simulink model "top_model"  (R2017a)
settings: Solver=VariableStepAuto  StartTime=0.0  StopTime=10.0  RelTol=1e-3  EnableMultiTasking=on
PostLoadFcn:
  | load('pcoeffs.mat');
  | load('rcoeffs.mat');
  | 
  | %load('purelongdata.mat');
  | %load('purelongdataval.mat');
  | %load('purelatdata.mat');
  | %load('purelatdataval.mat');
  | load('combineddata.mat');
undefined symbols (not defined in the file): p_Cx1, p_Cy1, p_Dx1, p_Dx2, p_Dx3, p_Dy1, p_Dy2, p_Dy3, p_Ex1, p_Ex2, p_Ex3, p_Ex4, p_Ey1, p_Ey2, p_Ey3, p_Ey4, p_Ey5, p_Kx1, p_Kx2, p_Kx3, p_Ky1, p_Ky2, p_Ky3, p_Ky4, p_Ky5, p_px1, p_px2, p_px3, p_px4, p_py1, p_py2, p_py3, p_py4, r_Bx1, r_Bx2, r_Bx3, r_By1, r_By2, r_By3, r_By4, r_Cx1, r_Cy1, r_Ex1, r_Ex2, r_Ey1, r_Ey2, r_Hx1, r_Hy1, r_Hy2, r_Vy1, r_Vy2, r_Vy3, r_Vy4, r_Vy5, r_Vy6
libraries: simulink_extras x2
settings Model: Creator=The MathWorks, Inc.  LastModifiedBy=Jianming
settings DataIOCC: LimitDataPoints=on
settings OptimizationCC: LifeSpan=inf
settings DebuggingCC: AllowSymbolicDim=off  SFUnexpectedBacktrackingDiag=warning  SFNoUnconditionalDefaultTransitionDiag=warning  SFExecutionAtInitializationDiag=none
settings ModelReferenceCC: PropagateSignalLabelsOutOfModel=off
settings GRTTargetCC: TargetLangStandard=C89/C90 (ANSI)
settings ConfigComp: CovMetricSettings=dw  CovHtmlReporting=on  CovSaveCumulativeToWorkspaceVar=on  CovSaveSingleToWorkspaceVar=on  CovExternalEMLEnable=off

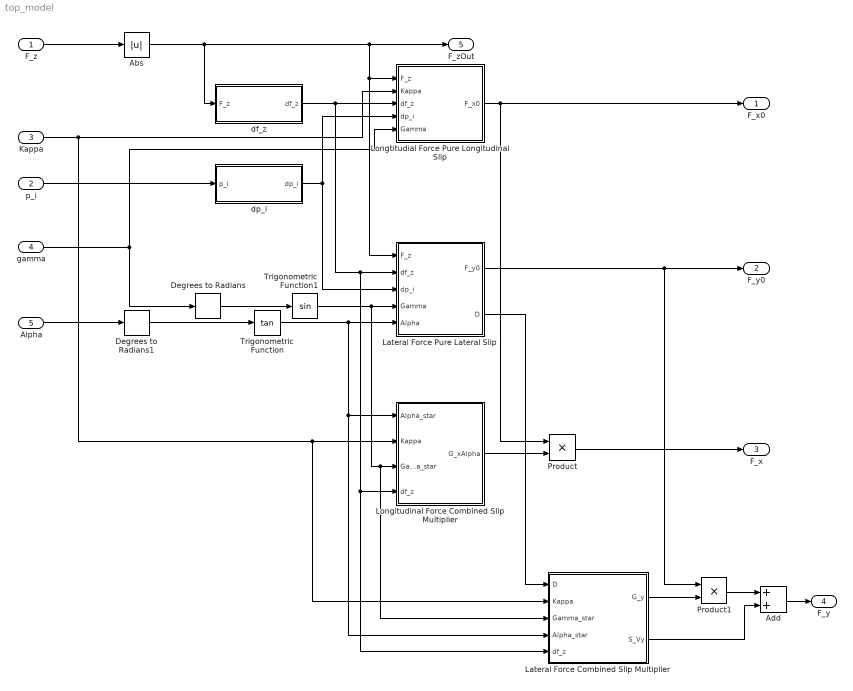
== system top_model ==
  F_z : Inport
  p_i : Inport  Port=2
  Kappa : Inport  Port=3
  gamma : Inport  Port=4
  Alpha : Inport  Port=5
  Abs : Abs
  Add : Sum
  Degrees to Radians : simulink_extras/Transformations/Degrees to Radians
  Degrees to Radians1 : simulink_extras/Transformations/Degrees to Radians
  Lateral Force Combined Slip Multiplier : Subsystem
  Lateral Force Pure Lateral Slip : Subsystem
  Longitudinal Force Combined Slip Multiplier : Subsystem
  Longtitudial Force Pure Longitudinal Slip : Subsystem
  Product : Product
  Product1 : Product
  Trigonometric Function : Trigonometry  Operator=tan
  Trigonometric Function1 : Trigonometry
  df_z : Subsystem
  dp_i : Subsystem
  F_x0 : Outport
  F_y0 : Outport  Port=2
  F_x : Outport  Port=3
  F_y : Outport  Port=4
  F_zOut : Outport  Port=5
  wires:
  Longtitudial Force Pure Longitudinal Slip/1(F_x0) -> Product/1, F_x0/1
  df_z/1(df_z) -> Lateral Force Combined Slip Multiplier/5(df_z), Longitudinal Force Combined Slip Multiplier/4(df_z), Lateral Force Pure Lateral Slip/2(df_z), Longtitudial Force Pure Longitudinal Slip/3(df_z)
  dp_i/1(dp_i) -> Lateral Force Pure Lateral Slip/3(dp_i), Longtitudial Force Pure Longitudinal Slip/4(dp_i)
  gamma/1 -> Longtitudial Force Pure Longitudinal Slip/5(Gamma), Degrees to Radians/1
  Kappa/1 -> Lateral Force Combined Slip Multiplier/2(Kappa), Longitudinal Force Combined Slip Multiplier/2(Kappa), Longtitudial Force Pure Longitudinal Slip/2(Kappa)
  p_i/1 -> dp_i/1(p_i)
  Lateral Force Pure Lateral Slip/1(F_y0) -> Product1/1, F_y0/1
  Alpha/1 -> Degrees to Radians1/1
  Degrees to Radians/1 -> Trigonometric Function1/1
  Degrees to Radians1/1 -> Trigonometric Function/1
  Trigonometric Function/1 -> Lateral Force Combined Slip Multiplier/4(Alpha_star), Longitudinal Force Combined Slip Multiplier/1(Alpha_star), Lateral Force Pure Lateral Slip/5(Alpha)
  Trigonometric Function1/1 -> Lateral Force Combined Slip Multiplier/3(Gamma_star), Longitudinal Force Combined Slip Multiplier/3(Gamma_star), Lateral Force Pure Lateral Slip/4(Gamma)
  F_z/1 -> Abs/1
  Longitudinal Force Combined Slip Multiplier/1(G_xAlpha) -> Product/2
  Product/1 -> F_x/1
  Lateral Force Pure Lateral Slip/2(D) -> Lateral Force Combined Slip Multiplier/1(D)
  Lateral Force Combined Slip Multiplier/1(G_y) -> Product1/2
  Abs/1 -> df_z/1(F_z), F_zOut/1, Lateral Force Pure Lateral Slip/1(F_z), Longtitudial Force Pure Longitudinal Slip/1(F_z)
  Product1/1 -> Add/1
  Lateral Force Combined Slip Multiplier/2(S_Vy) -> Add/2
  Add/1 -> F_y/1

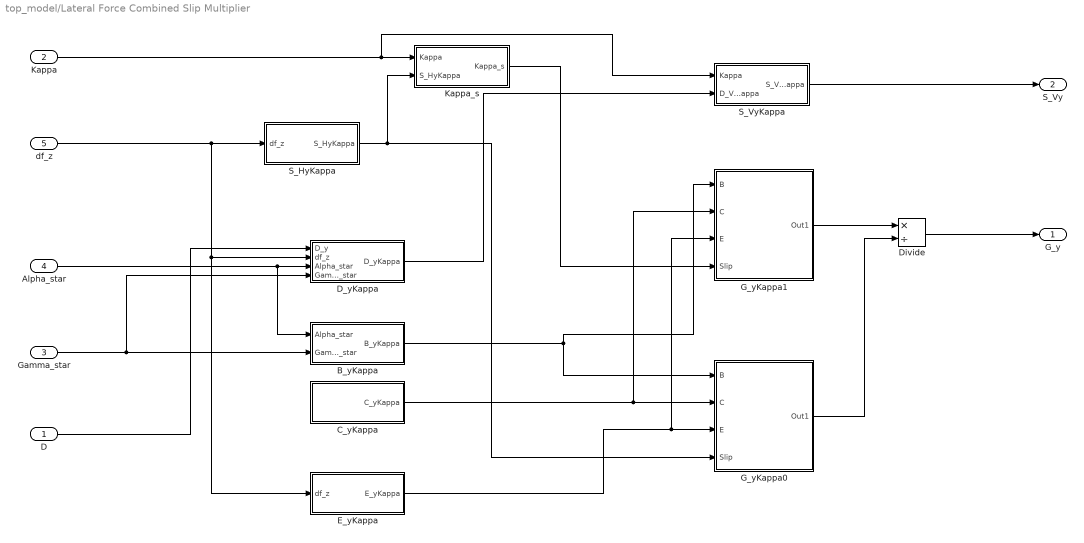
== system top_model/Lateral Force Combined Slip Multiplier ==
  D : Inport
  Kappa : Inport  Port=2
  Gamma_star : Inport  Port=3
  Alpha_star : Inport  Port=4
  df_z : Inport  Port=5
  B_yKappa : Subsystem
  C_yKappa : Subsystem
  D_yKappa : Subsystem
  Divide : Product  Inputs=*/
  E_yKappa : Subsystem
  G_yKappa0 : Subsystem
  G_yKappa1 : Subsystem
  Kappa_s : Subsystem
  S_HyKappa : Subsystem
  S_VyKappa : Subsystem
  G_y : Outport
  S_Vy : Outport  Port=2
  wires:
  G_yKappa1/1(Out1) -> Divide/1
  G_yKappa0/1(Out1) -> Divide/2
  S_VyKappa/1(S_VyKappa) -> S_Vy/1
  Divide/1 -> G_y/1
  Kappa/1 -> S_VyKappa/1(Kappa), Kappa_s/1(Kappa)
  S_HyKappa/1(S_HyKappa) -> Kappa_s/2(S_HyKappa), G_yKappa0/4(Slip)
  df_z/1 -> E_yKappa/1(df_z), D_yKappa/2(df_z), S_HyKappa/1(df_z)
  Kappa_s/1(Kappa_s) -> G_yKappa1/4(Slip)
  C_yKappa/1(C_yKappa) -> G_yKappa1/2(C), G_yKappa0/2(C)
  E_yKappa/1(E_yKappa) -> G_yKappa1/3(E), G_yKappa0/3(E)
  D/1 -> D_yKappa/1(D_y)
  Alpha_star/1 -> B_yKappa/1(Alpha_star), D_yKappa/3(Alpha_star)
  Gamma_star/1 -> D_yKappa/4(Gamma_star), B_yKappa/2(Gamma_star)
  D_yKappa/1(D_yKappa) -> S_VyKappa/2(D_VyKappa)
  B_yKappa/1(B_yKappa) -> G_yKappa1/1(B), G_yKappa0/1(B)

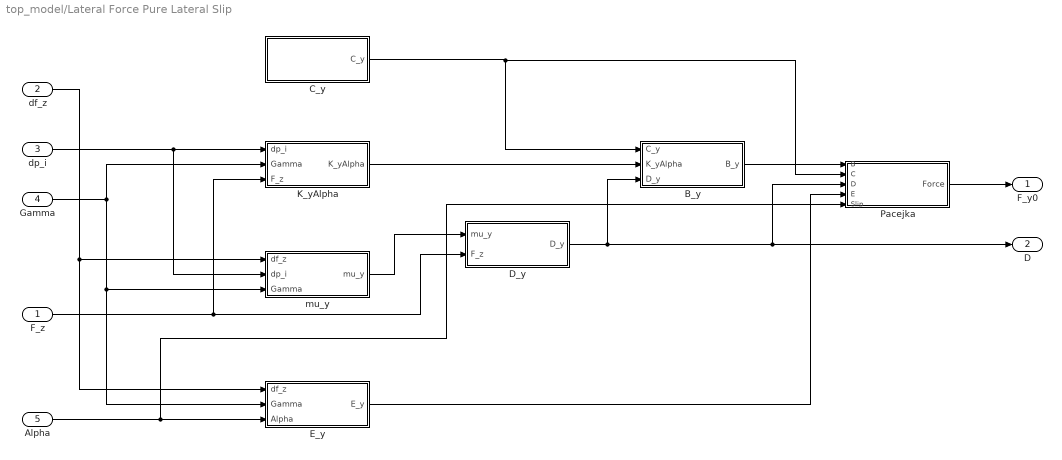
== system top_model/Lateral Force Pure Lateral Slip ==
  F_z : Inport
  df_z : Inport  Port=2
  dp_i : Inport  Port=3
  Gamma : Inport  Port=4
  Alpha : Inport  Port=5
  B_y : Subsystem
  C_y : Subsystem
  D_y : Subsystem
  E_y : Subsystem
  K_yAlpha : Subsystem
  Pacejka : Subsystem
  mu_y : Subsystem
  F_y0 : Outport
  D : Outport  Port=2
  wires:
  K_yAlpha/1(K_yAlpha) -> B_y/2(K_yAlpha)
  Pacejka/1(Force) -> F_y0/1
  D_y/1(D_y) -> D/1, Pacejka/3(D), B_y/3(D_y)
  C_y/1(C_y) -> Pacejka/2(C), B_y/1(C_y)
  B_y/1(B_y) -> Pacejka/1(B)
  E_y/1(E_y) -> Pacejka/4(E)
  mu_y/1(mu_y) -> D_y/1(mu_y)
  F_z/1 -> K_yAlpha/3(F_z), D_y/2(F_z)
  Alpha/1 -> E_y/3(Alpha), Pacejka/5("Slip ")
  df_z/1 -> E_y/1(df_z), mu_y/1(df_z)
  dp_i/1 -> mu_y/2(dp_i), K_yAlpha/1(dp_i)
  Gamma/1 -> E_y/2(Gamma), mu_y/3(Gamma), K_yAlpha/2(Gamma)

== system top_model/Longitudinal Force Combined Slip Multiplier ==
  Alpha_star : Inport
  Kappa : Inport  Port=2
  Gamma_star : Inport  Port=3
  df_z : Inport  Port=4
  Alpha_s : Subsystem
  B_xAlpha : Subsystem
  C_xAlpha : Subsystem
  Divide : Product  Inputs=*/
  E_xAlpha : Subsystem
  G_xAlpha0 : Subsystem
  G_xAlpha2 : Subsystem
  S_HxAlpha : Subsystem
  G_xAlpha : Outport
  wires:
  Alpha_star/1 -> Alpha_s/1(Alpha_star)
  S_HxAlpha/1(S_HxAlpha) -> G_xAlpha0/4(Slip), Alpha_s/2(S_HxAlpha)
  df_z/1 -> E_xAlpha/1(df_z)
  Kappa/1 -> B_xAlpha/2(Kappa)
  Gamma_star/1 -> B_xAlpha/1(Gamma_star)
  B_xAlpha/1(B_xAlpha) -> G_xAlpha0/1(B), G_xAlpha2/1(B)
  C_xAlpha/1(C_xAlpha) -> G_xAlpha0/2(C), G_xAlpha2/2(C)
  E_xAlpha/1(E_xAlpha) -> G_xAlpha0/3(E), G_xAlpha2/3(E)
  Alpha_s/1(Alpha_s) -> G_xAlpha2/4(Slip)
  G_xAlpha2/1(Out1) -> Divide/1
  G_xAlpha0/1(Out1) -> Divide/2
  Divide/1 -> G_xAlpha/1

== system top_model/Longtitudial Force Pure Longitudinal Slip ==
  F_z : Inport
  Kappa : Inport  Port=2
  df_z : Inport  Port=3
  dp_i : Inport  Port=4
  Gamma : Inport  Port=5
  B_x : Subsystem
  "C_x " : Subsystem
  D_x : Subsystem
  E_x : Subsystem
  K_xKappa : Subsystem
  Pacejka : Subsystem
  mu_x : Subsystem
  F_x0 : Outport
  wires:
  mu_x/1(mu_x) -> D_x/2(mu_x)
  F_z/1 -> K_xKappa/1(F_z), D_x/1(F_z)
  D_x/1(D_x) -> Pacejka/3(D), B_x/3(D_x)
  "C_x "/1(C_x) -> Pacejka/2(C), B_x/1(C_x)
  K_xKappa/1(K_xKappa) -> B_x/2(K_xKappa)
  E_x/1(E_x) -> Pacejka/4(E)
  B_x/1(B_x) -> Pacejka/1(B)
  Pacejka/1(Force) -> F_x0/1
  df_z/1 -> K_xKappa/2(df_z), E_x/1(df_z), mu_x/1(df_z)
  dp_i/1 -> K_xKappa/3(dp_i), mu_x/2(dp_i)
  Gamma/1 -> mu_x/3(Gamma)
  Kappa/1 -> E_x/2("kappa "), Pacejka/5("Slip ")

== system top_model/df_z ==
  F_z : Inport
  Divide : Product  Inputs=*/
  F_z0 : Constant  Value=250 * 4.448
  Subtract : Sum  Inputs=+-
  df_z : Outport
  wires:
  F_z/1 -> Subtract/1
  Subtract/1 -> Divide/1
  F_z0/1 -> Divide/2, Subtract/2
  Divide/1 -> df_z/1

== system top_model/dp_i ==
  p_i : Inport
  Divide : Product  Inputs=*/
  Subtract : Sum  Inputs=+-
  p_i0 : Constant  Value=12 * 6.89476
  dp_i : Outport
  wires:
  p_i/1 -> Subtract/1
  Subtract/1 -> Divide/1
  Divide/1 -> dp_i/1
  p_i0/1 -> Divide/2, Subtract/2

== system top_model/Lateral Force Combined Slip Multiplier/B_yKappa ==
  Alpha_star : Inport
  Gamma_star : Inport  Port=2
  Add : Sum
  Constant : Constant  Value=r_By1
  Constant1 : Constant  Value=r_By2
  Constant2 : Constant  Value=r_By3
  Constant3 : Constant  Value=r_By4
  Cos : Trigonometry  Operator=cos
  Product : Product
  Product1 : Product  Inputs=3
  Product2 : Product
  Subtract : Sum  Inputs=+-
  atan : Trigonometry  Operator=atan
  B_yKappa : Outport
  wires:
  Alpha_star/1 -> Subtract/1
  Constant2/1 -> Subtract/2
  Subtract/1 -> Product/2
  Constant1/1 -> Product/1
  Product/1 -> atan/1
  atan/1 -> Cos/1
  Gamma_star/1 -> Product1/2, Product1/1
  Constant3/1 -> Product1/3
  Product1/1 -> Add/2
  Constant/1 -> Add/1
  Cos/1 -> Product2/1
  Add/1 -> Product2/2
  Product2/1 -> B_yKappa/1

== system top_model/Lateral Force Combined Slip Multiplier/C_yKappa ==
  Constant : Constant  Value=r_Cy1
  C_yKappa : Outport
  wires:
  Constant/1 -> C_yKappa/1

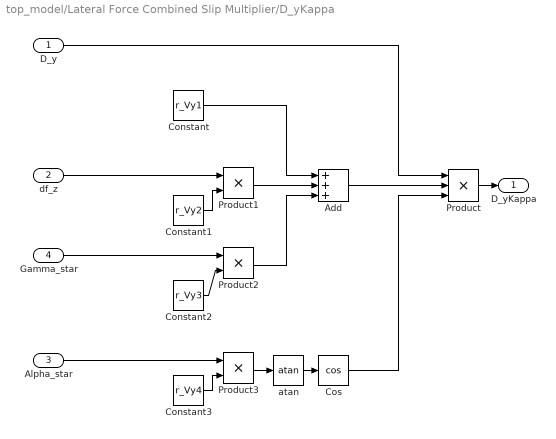
== system top_model/Lateral Force Combined Slip Multiplier/D_yKappa ==
  D_y : Inport
  df_z : Inport  Port=2
  Alpha_star : Inport  Port=3
  Gamma_star : Inport  Port=4
  Add : Sum  Inputs=3
  Constant : Constant  Value=r_Vy1
  Constant1 : Constant  Value=r_Vy2
  Constant2 : Constant  Value=r_Vy3
  Constant3 : Constant  Value=r_Vy4
  Cos : Trigonometry  Operator=cos
  Product : Product  Inputs=3
  Product1 : Product
  Product2 : Product
  Product3 : Product
  atan : Trigonometry  Operator=atan
  D_yKappa : Outport
  wires:
  Product/1 -> D_yKappa/1
  df_z/1 -> Product1/1
  Constant1/1 -> Product1/2
  Constant2/1 -> Product2/2
  Gamma_star/1 -> Product2/1
  Alpha_star/1 -> Product3/1
  Constant3/1 -> Product3/2
  Product3/1 -> atan/1
  atan/1 -> Cos/1
  Constant/1 -> Add/1
  Product1/1 -> Add/2
  Product2/1 -> Add/3
  Add/1 -> Product/2
  Cos/1 -> Product/3
  D_y/1 -> Product/1

== system top_model/Lateral Force Combined Slip Multiplier/E_yKappa ==
  df_z : Inport
  Add : Sum
  Constant : Constant  Value=r_Ey1
  Constant1 : Constant  Value=r_Ey2
  Constant2 : Constant
  Min : MinMax  Inputs=2
  Product : Product
  E_yKappa : Outport
  wires:
  df_z/1 -> Product/1
  Constant1/1 -> Product/2
  Product/1 -> Add/2
  Constant/1 -> Add/1
  Add/1 -> Min/1
  Constant2/1 -> Min/2
  Min/1 -> E_yKappa/1

== system top_model/Lateral Force Combined Slip Multiplier/G_yKappa0 ==
  B : Inport
  C : Inport  Port=2
  E : Inport  Port=3
  Slip : Inport  Port=4
  Cos : Trigonometry  Operator=cos
  Product : Product
  Product1 : Product
  Product2 : Product
  Subtract : Sum  Inputs=+-
  Subtract1 : Sum  Inputs=+-
  atan : Trigonometry  Operator=atan
  atan1 : Trigonometry  Operator=atan
  Out1 : Outport
  wires:
  B/1 -> Product/2
  Slip/1 -> Product/1
  Product/1 -> Subtract1/1, Subtract/1, atan/1
  atan/1 -> Subtract/2
  Subtract/1 -> Product1/1
  E/1 -> Product1/2
  Product1/1 -> Subtract1/2
  Subtract1/1 -> atan1/1
  atan1/1 -> Product2/1
  C/1 -> Product2/2
  Product2/1 -> Cos/1
  Cos/1 -> Out1/1

== system top_model/Lateral Force Combined Slip Multiplier/G_yKappa1 ==
  B : Inport
  C : Inport  Port=2
  E : Inport  Port=3
  Slip : Inport  Port=4
  Cos : Trigonometry  Operator=cos
  Product : Product
  Product1 : Product
  Product2 : Product
  Subtract : Sum  Inputs=+-
  Subtract1 : Sum  Inputs=+-
  atan : Trigonometry  Operator=atan
  atan1 : Trigonometry  Operator=atan
  Out1 : Outport
  wires:
  B/1 -> Product/2
  Slip/1 -> Product/1
  Product/1 -> Subtract1/1, Subtract/1, atan/1
  atan/1 -> Subtract/2
  Subtract/1 -> Product1/1
  E/1 -> Product1/2
  Product1/1 -> Subtract1/2
  Subtract1/1 -> atan1/1
  atan1/1 -> Product2/1
  C/1 -> Product2/2
  Product2/1 -> Cos/1
  Cos/1 -> Out1/1

== system top_model/Lateral Force Combined Slip Multiplier/Kappa_s ==
  Kappa : Inport
  S_HyKappa : Inport  Port=2
  Add : Sum
  Kappa_s : Outport
  wires:
  Kappa/1 -> Add/1
  S_HyKappa/1 -> Add/2
  Add/1 -> Kappa_s/1

== system top_model/Lateral Force Combined Slip Multiplier/S_HyKappa ==
  df_z : Inport
  Add : Sum
  Constant : Constant  Value=r_Hy1
  Constant1 : Constant  Value=r_Hy2
  Product : Product
  S_HyKappa : Outport
  wires:
  df_z/1 -> Product/1
  Constant1/1 -> Product/2
  Product/1 -> Add/2
  Constant/1 -> Add/1
  Add/1 -> S_HyKappa/1

== system top_model/Lateral Force Combined Slip Multiplier/S_VyKappa ==
  Kappa : Inport
  D_VyKappa : Inport  Port=2
  Constant : Constant  Value=r_Vy5
  Constant1 : Constant  Value=r_Vy6
  Product : Product
  Product1 : Product
  Product2 : Product
  Sin : Trigonometry
  atan : Trigonometry  Operator=atan
  S_VyKappa : Outport
  wires:
  Kappa/1 -> Product/1
  Constant1/1 -> Product/2
  Product/1 -> atan/1
  atan/1 -> Product1/2
  Constant/1 -> Product1/1
  Product1/1 -> Sin/1
  Sin/1 -> Product2/1
  D_VyKappa/1 -> Product2/2
  Product2/1 -> S_VyKappa/1

== system top_model/Lateral Force Pure Lateral Slip/B_y ==
  C_y : Inport
  K_yAlpha : Inport  Port=2
  D_y : Inport  Port=3
  Add : Sum
  Divide : Product  Inputs=*/
  Product : Product
  "epsilon " : Constant  Value=0.001
  B_y : Outport
  wires:
  C_y/1 -> Product/1
  D_y/1 -> Product/2
  Product/1 -> Add/1
  "epsilon "/1 -> Add/2
  K_yAlpha/1 -> Divide/1
  Add/1 -> Divide/2
  Divide/1 -> B_y/1

== system top_model/Lateral Force Pure Lateral Slip/C_y ==
  Constant : Constant  Value=p_Cy1
  Constant1 : Constant  Value=0
  Min : MinMax  Function=max  Inputs=2
  C_y : Outport
  wires:
  Constant/1 -> Min/1
  Constant1/1 -> Min/2
  Min/1 -> C_y/1

== system top_model/Lateral Force Pure Lateral Slip/D_y ==
  mu_y : Inport
  F_z : Inport  Port=2
  Constant : Constant  Value=-1000000
  Min : MinMax  Function=max  Inputs=2
  Product : Product
  D_y : Outport
  wires:
  mu_y/1 -> Product/1
  F_z/1 -> Product/2
  Min/1 -> D_y/1
  Product/1 -> Min/1
  Constant/1 -> Min/2

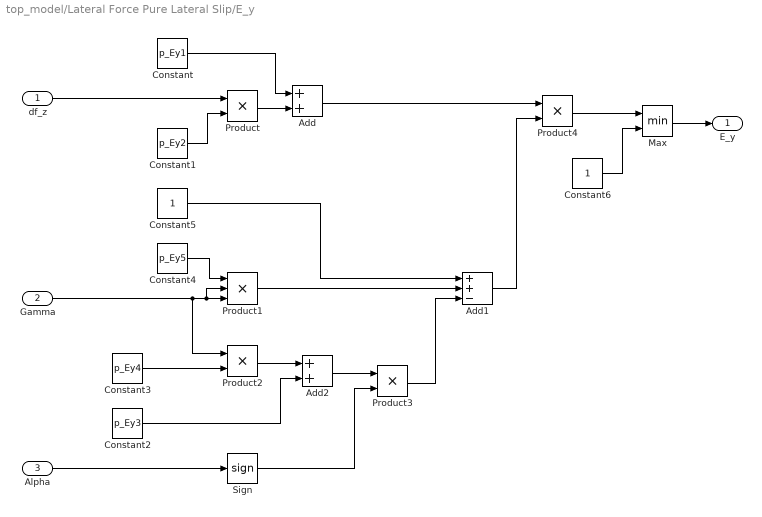
== system top_model/Lateral Force Pure Lateral Slip/E_y ==
  df_z : Inport
  Gamma : Inport  Port=2
  Alpha : Inport  Port=3
  Add : Sum
  Add1 : Sum  Inputs=++-
  Add2 : Sum
  Constant : Constant  Value=p_Ey1
  Constant1 : Constant  Value=p_Ey2
  Constant2 : Constant  Value=p_Ey3
  Constant3 : Constant  Value=p_Ey4
  Constant4 : Constant  Value=p_Ey5
  Constant5 : Constant
  Constant6 : Constant
  Max : MinMax  Inputs=2
  Product{,2..4} (4 alike) : Product
  Product1 : Product  Inputs=3
  Sign : Signum
  E_y : Outport
  wires:
  df_z/1 -> Product/1
  Constant1/1 -> Product/2
  Product/1 -> Add/2
  Constant/1 -> Add/1
  Constant4/1 -> Product1/1
  Gamma/1 -> Product2/1, Product1/2, Product1/3
  Product1/1 -> Add1/2
  Constant5/1 -> Add1/1
  Constant3/1 -> Product2/2
  Product2/1 -> Add2/1
  Constant2/1 -> Add2/2
  Add2/1 -> Product3/1
  Alpha/1 -> Sign/1
  Sign/1 -> Product3/2
  Product3/1 -> Add1/3
  Add/1 -> Product4/1
  Add1/1 -> Product4/2
  Product4/1 -> Max/1
  Constant6/1 -> Max/2
  Max/1 -> E_y/1

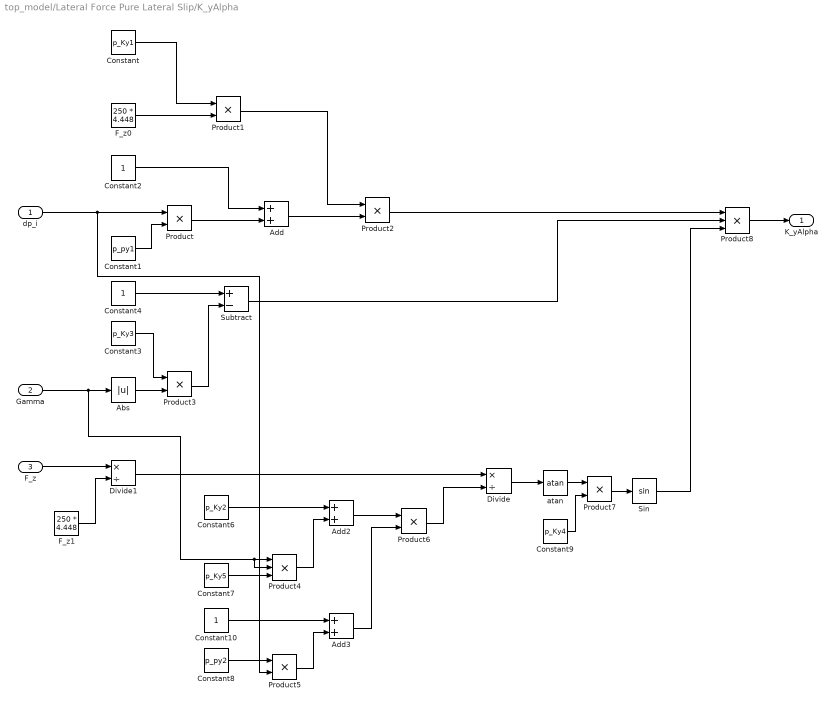
== system top_model/Lateral Force Pure Lateral Slip/K_yAlpha ==
  dp_i : Inport
  Gamma : Inport  Port=2
  F_z : Inport  Port=3
  Abs : Abs
  Add : Sum
  Add2 : Sum
  Add3 : Sum
  Constant : Constant  Value=p_Ky1
  Constant1 : Constant  Value=p_py1
  Constant10 : Constant
  Constant2 : Constant
  Constant3 : Constant  Value=p_Ky3
  Constant4 : Constant
  Constant6 : Constant  Value=p_Ky2
  Constant7 : Constant  Value=p_Ky5
  Constant8 : Constant  Value=p_py2
  Constant9 : Constant  Value=p_Ky4
  Divide : Product  Inputs=*/
  Divide1 : Product  Inputs=*/
  F_z0 : Constant  Value=250 * 4.448
  F_z1 : Constant  Value=250 * 4.448
  Product{,1..3,5..7} (7 alike) : Product
  Product4 : Product  Inputs=3
  Product8 : Product  Inputs=3
  Sin : Trigonometry
  Subtract : Sum  Inputs=+-
  atan : Trigonometry  Operator=atan
  K_yAlpha : Outport
  wires:
  dp_i/1 -> Product5/2, Product/1
  Constant1/1 -> Product/2
  Product/1 -> Add/2
  Constant2/1 -> Add/1
  F_z0/1 -> Product1/2
  Constant/1 -> Product1/1
  Add/1 -> Product2/2
  Product1/1 -> Product2/1
  Constant4/1 -> Subtract/1
  Gamma/1 -> Product4/1, Product4/2, Abs/1
  Constant3/1 -> Product3/1
  Product3/1 -> Subtract/2
  Abs/1 -> Product3/2
  Constant7/1 -> Product4/3
  Product4/1 -> Add2/2
  Constant6/1 -> Add2/1
  Constant8/1 -> Product5/1
  Add2/1 -> Product6/1
  Product6/1 -> Divide/2
  Divide1/1 -> Divide/1
  Divide/1 -> atan/1
  atan/1 -> Product7/1
  Constant9/1 -> Product7/2
  Product7/1 -> Sin/1
  Product2/1 -> Product8/1
  Subtract/1 -> Product8/2
  Sin/1 -> Product8/3
  Product8/1 -> K_yAlpha/1
  Constant10/1 -> Add3/1
  Product5/1 -> Add3/2
  Add3/1 -> Product6/2
  F_z1/1 -> Divide1/2
  F_z/1 -> Divide1/1

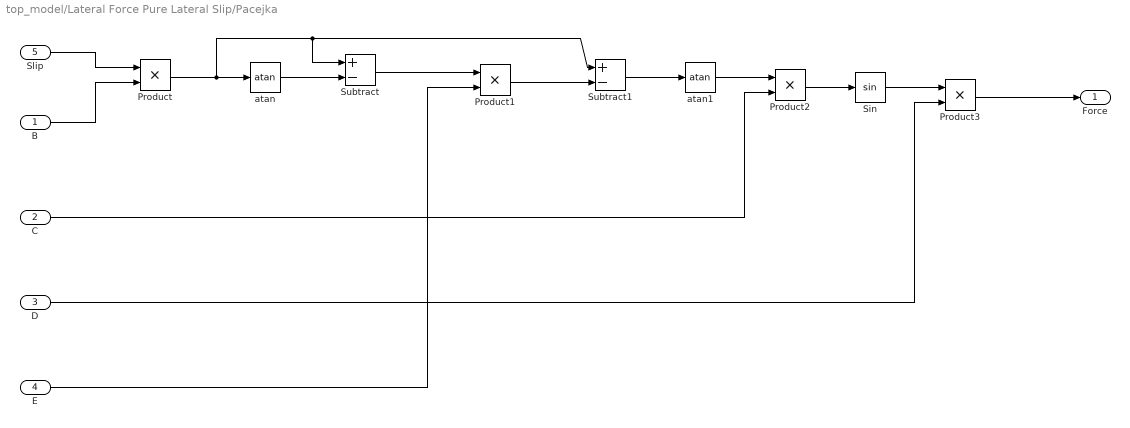
== system top_model/Lateral Force Pure Lateral Slip/Pacejka ==
  B : Inport
  C : Inport  Port=2
  D : Inport  Port=3
  E : Inport  Port=4
  "Slip " : Inport  Port=5
  Product{,1..3} (4 alike) : Product
  Sin : Trigonometry
  Subtract : Sum  Inputs=+-
  Subtract1 : Sum  Inputs=+-
  atan : Trigonometry  Operator=atan
  atan1 : Trigonometry  Operator=atan
  Force : Outport
  wires:
  "Slip "/1 -> Product/1
  B/1 -> Product/2
  Product/1 -> Subtract1/1, Subtract/1, atan/1
  atan/1 -> Subtract/2
  Subtract/1 -> Product1/1
  E/1 -> Product1/2
  Product1/1 -> Subtract1/2
  Subtract1/1 -> atan1/1
  atan1/1 -> Product2/1
  C/1 -> Product2/2
  Product2/1 -> Sin/1
  Sin/1 -> Product3/1
  D/1 -> Product3/2
  Product3/1 -> Force/1

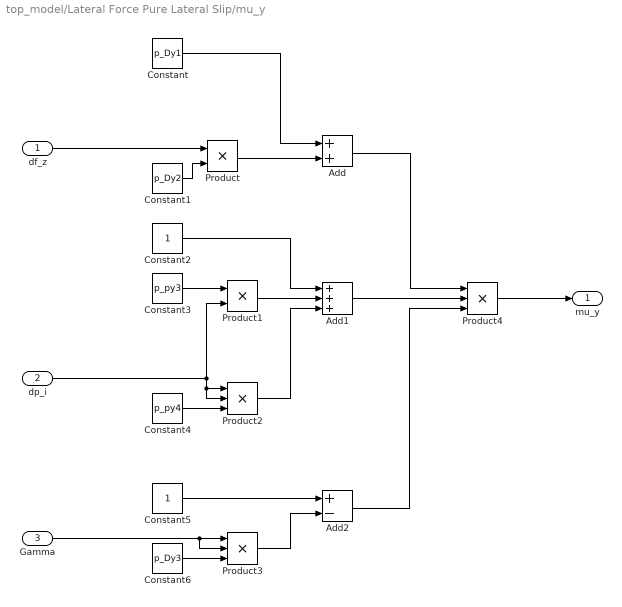
== system top_model/Lateral Force Pure Lateral Slip/mu_y ==
  df_z : Inport
  dp_i : Inport  Port=2
  Gamma : Inport  Port=3
  Add : Sum
  Add1 : Sum  Inputs=3
  Add2 : Sum  Inputs=+-
  Constant : Constant  Value=p_Dy1
  Constant1 : Constant  Value=p_Dy2
  Constant2 : Constant
  Constant3 : Constant  Value=p_py3
  Constant4 : Constant  Value=p_py4
  Constant5 : Constant
  Constant6 : Constant  Value=p_Dy3
  Product : Product
  Product1 : Product
  Product2 : Product  Inputs=3
  Product3 : Product  Inputs=3
  Product4 : Product  Inputs=3
  mu_y : Outport
  wires:
  df_z/1 -> Product/1
  Constant1/1 -> Product/2
  Product/1 -> Add/2
  Constant/1 -> Add/1
  Constant3/1 -> Product1/1
  dp_i/1 -> Product2/1, Product2/2, Product1/2
  Constant4/1 -> Product2/3
  Product1/1 -> Add1/2
  Constant2/1 -> Add1/1
  Product2/1 -> Add1/3
  Gamma/1 -> Product3/2, Product3/1
  Constant6/1 -> Product3/3
  Constant5/1 -> Add2/1
  Product3/1 -> Add2/2
  Add1/1 -> Product4/2
  Add/1 -> Product4/1
  Add2/1 -> Product4/3
  Product4/1 -> mu_y/1

== system top_model/Longitudinal Force Combined Slip Multiplier/Alpha_s ==
  Alpha_star : Inport
  S_HxAlpha : Inport  Port=2
  Add : Sum
  Alpha_s : Outport
  wires:
  Alpha_star/1 -> Add/1
  S_HxAlpha/1 -> Add/2
  Add/1 -> Alpha_s/1

== system top_model/Longitudinal Force Combined Slip Multiplier/B_xAlpha ==
  Gamma_star : Inport
  Kappa : Inport  Port=2
  Add : Sum
  Constant : Constant  Value=r_Bx1
  Constant1 : Constant  Value=r_Bx2
  Constant2 : Constant  Value=r_Bx3
  Constant3 : Constant  Value=0
  Cos : Trigonometry  Operator=cos
  Max : MinMax  Function=max  Inputs=2
  Product : Product  Inputs=3
  Product1 : Product
  Product2 : Product
  atan : Trigonometry  Operator=atan
  B_xAlpha : Outport
  wires:
  Gamma_star/1 -> Product/2, Product/1
  Constant2/1 -> Product/3
  Product/1 -> Add/2
  Constant/1 -> Add/1
  Kappa/1 -> Product1/1
  Constant1/1 -> Product1/2
  Product1/1 -> atan/1
  atan/1 -> Cos/1
  Add/1 -> Product2/1
  Cos/1 -> Product2/2
  Product2/1 -> Max/1
  Constant3/1 -> Max/2
  Max/1 -> B_xAlpha/1

== system top_model/Longitudinal Force Combined Slip Multiplier/C_xAlpha ==
  Constant : Constant  Value=r_Cx1
  C_xAlpha : Outport
  wires:
  Constant/1 -> C_xAlpha/1

== system top_model/Longitudinal Force Combined Slip Multiplier/E_xAlpha ==
  df_z : Inport
  Add : Sum
  Constant : Constant  Value=r_Ex1
  Constant1 : Constant  Value=r_Ex2
  Constant2 : Constant
  Min : MinMax  Inputs=2
  Product : Product
  E_xAlpha : Outport
  wires:
  df_z/1 -> Product/1
  Constant1/1 -> Product/2
  Product/1 -> Add/2
  Constant/1 -> Add/1
  Add/1 -> Min/1
  Constant2/1 -> Min/2
  Min/1 -> E_xAlpha/1

== system top_model/Longitudinal Force Combined Slip Multiplier/G_xAlpha0 ==
  B : Inport
  C : Inport  Port=2
  E : Inport  Port=3
  Slip : Inport  Port=4
  Cos : Trigonometry  Operator=cos
  Product : Product
  Product1 : Product
  Product2 : Product
  Subtract : Sum  Inputs=+-
  Subtract1 : Sum  Inputs=+-
  atan : Trigonometry  Operator=atan
  atan1 : Trigonometry  Operator=atan
  Out1 : Outport
  wires:
  B/1 -> Product/2
  Slip/1 -> Product/1
  Product/1 -> Subtract1/1, Subtract/1, atan/1
  atan/1 -> Subtract/2
  Subtract/1 -> Product1/1
  E/1 -> Product1/2
  Product1/1 -> Subtract1/2
  Subtract1/1 -> atan1/1
  atan1/1 -> Product2/1
  C/1 -> Product2/2
  Product2/1 -> Cos/1
  Cos/1 -> Out1/1

== system top_model/Longitudinal Force Combined Slip Multiplier/G_xAlpha2 ==
  B : Inport
  C : Inport  Port=2
  E : Inport  Port=3
  Slip : Inport  Port=4
  Cos : Trigonometry  Operator=cos
  Product : Product
  Product1 : Product
  Product2 : Product
  Subtract : Sum  Inputs=+-
  Subtract1 : Sum  Inputs=+-
  atan : Trigonometry  Operator=atan
  atan1 : Trigonometry  Operator=atan
  Out1 : Outport
  wires:
  B/1 -> Product/2
  Slip/1 -> Product/1
  Product/1 -> Subtract1/1, Subtract/1, atan/1
  atan/1 -> Subtract/2
  Subtract/1 -> Product1/1
  E/1 -> Product1/2
  Product1/1 -> Subtract1/2
  Subtract1/1 -> atan1/1
  atan1/1 -> Product2/1
  C/1 -> Product2/2
  Product2/1 -> Cos/1
  Cos/1 -> Out1/1

== system top_model/Longitudinal Force Combined Slip Multiplier/S_HxAlpha ==
  Constant : Constant  Value=r_Hx1
  S_HxAlpha : Outport
  wires:
  Constant/1 -> S_HxAlpha/1

== system top_model/Longtitudial Force Pure Longitudinal Slip/B_x ==
  C_x : Inport
  K_xKappa : Inport  Port=2
  D_x : Inport  Port=3
  Add : Sum
  Constant : Constant  Value=0.001
  Divide : Product  Inputs=*/
  Product : Product
  B_x : Outport
  wires:
  C_x/1 -> Product/1
  D_x/1 -> Product/2
  Product/1 -> Add/1
  Constant/1 -> Add/2
  Add/1 -> Divide/2
  K_xKappa/1 -> Divide/1
  Divide/1 -> B_x/1

== system top_model/Longtitudial Force Pure Longitudinal Slip/C_x  ==
  Constant : Constant  Value=p_Cx1
  Constant1 : Constant  Value=0
  Max : MinMax  Function=max  Inputs=2
  C_x : Outport
  wires:
  Constant/1 -> Max/1
  Max/1 -> C_x/1
  Constant1/1 -> Max/2

== system top_model/Longtitudial Force Pure Longitudinal Slip/D_x ==
  F_z : Inport
  mu_x : Inport  Port=2
  Constant : Constant  Value=-100000
  Max : MinMax  Function=max  Inputs=2
  Product : Product
  D_x : Outport
  wires:
  F_z/1 -> Product/1
  mu_x/1 -> Product/2
  Max/1 -> D_x/1
  Product/1 -> Max/1
  Constant/1 -> Max/2

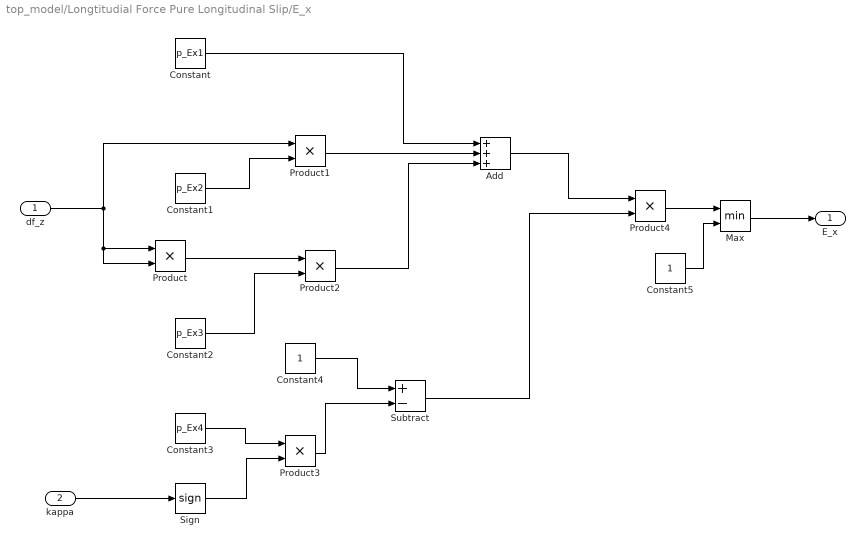
== system top_model/Longtitudial Force Pure Longitudinal Slip/E_x ==
  df_z : Inport
  "kappa " : Inport  Port=2
  Add : Sum  Inputs=3
  Constant : Constant  Value=p_Ex1
  Constant1 : Constant  Value=p_Ex2
  Constant2 : Constant  Value=p_Ex3
  Constant3 : Constant  Value=p_Ex4
  Constant4 : Constant
  Constant5 : Constant
  Max : MinMax  Inputs=2
  Product{,1..4} (5 alike) : Product
  Sign : Signum
  Subtract : Sum  Inputs=+-
  E_x : Outport
  wires:
  Product/1 -> Product2/1
  df_z/1 -> Product1/1, Product/2, Product/1
  Constant1/1 -> Product1/2
  Constant2/1 -> Product2/2
  Product1/1 -> Add/2
  Constant/1 -> Add/1
  Product2/1 -> Add/3
  "kappa "/1 -> Sign/1
  Constant3/1 -> Product3/1
  Sign/1 -> Product3/2
  Constant4/1 -> Subtract/1
  Product3/1 -> Subtract/2
  Add/1 -> Product4/1
  Subtract/1 -> Product4/2
  Product4/1 -> Max/1
  Constant5/1 -> Max/2
  Max/1 -> E_x/1

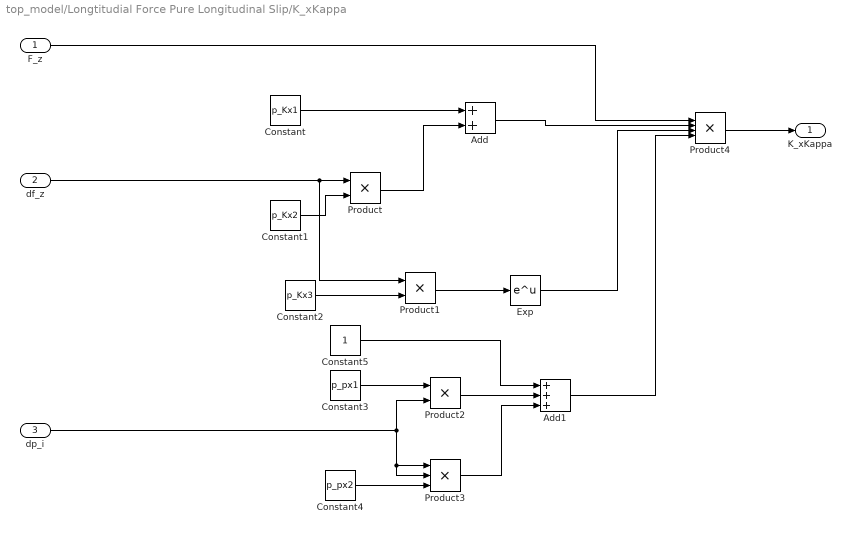
== system top_model/Longtitudial Force Pure Longitudinal Slip/K_xKappa ==
  F_z : Inport
  df_z : Inport  Port=2
  dp_i : Inport  Port=3
  Add : Sum
  Add1 : Sum  Inputs=3
  Constant : Constant  Value=p_Kx1
  Constant1 : Constant  Value=p_Kx2
  Constant2 : Constant  Value=p_Kx3
  Constant3 : Constant  Value=p_px1
  Constant4 : Constant  Value=p_px2
  Constant5 : Constant
  Exp : Math  SaturateOnIntegerOverflow=on
  Product : Product
  Product1 : Product
  Product2 : Product
  Product3 : Product  Inputs=3
  Product4 : Product  Inputs=4
  K_xKappa : Outport
  wires:
  df_z/1 -> Product1/1, Product/1
  Constant1/1 -> Product/2
  Constant/1 -> Add/1
  Product/1 -> Add/2
  Constant2/1 -> Product1/2
  Product1/1 -> Exp/1
  Constant3/1 -> Product2/1
  dp_i/1 -> Product3/1, Product3/2, Product2/2
  Constant4/1 -> Product3/3
  Product2/1 -> Add1/2
  Constant5/1 -> Add1/1
  Product3/1 -> Add1/3
  F_z/1 -> Product4/1
  Add/1 -> Product4/2
  Exp/1 -> Product4/3
  Add1/1 -> Product4/4
  Product4/1 -> K_xKappa/1

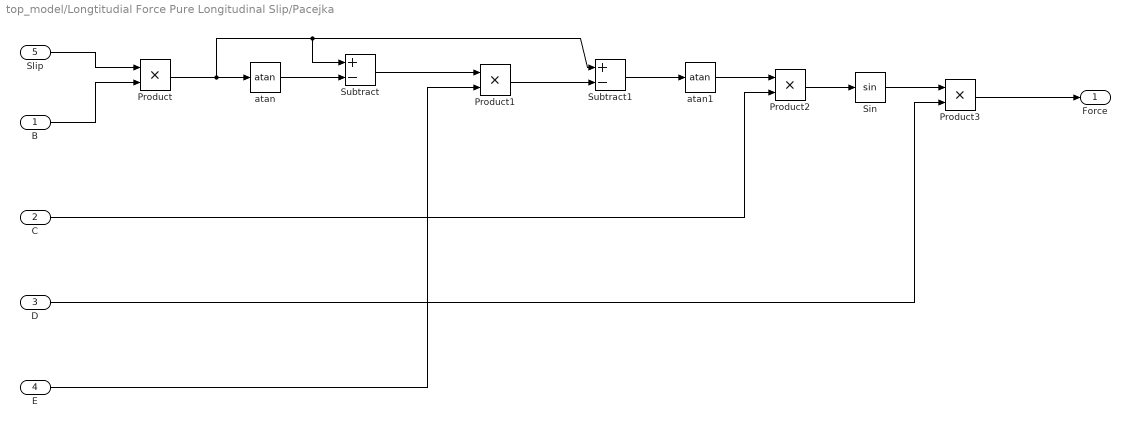
== system top_model/Longtitudial Force Pure Longitudinal Slip/Pacejka ==
  B : Inport
  C : Inport  Port=2
  D : Inport  Port=3
  E : Inport  Port=4
  "Slip " : Inport  Port=5
  Product{,1..3} (4 alike) : Product
  Sin : Trigonometry
  Subtract : Sum  Inputs=+-
  Subtract1 : Sum  Inputs=+-
  atan : Trigonometry  Operator=atan
  atan1 : Trigonometry  Operator=atan
  Force : Outport
  wires:
  "Slip "/1 -> Product/1
  B/1 -> Product/2
  Product/1 -> Subtract1/1, Subtract/1, atan/1
  atan/1 -> Subtract/2
  Subtract/1 -> Product1/1
  E/1 -> Product1/2
  Product1/1 -> Subtract1/2
  Subtract1/1 -> atan1/1
  atan1/1 -> Product2/1
  C/1 -> Product2/2
  Product2/1 -> Sin/1
  Sin/1 -> Product3/1
  D/1 -> Product3/2
  Product3/1 -> Force/1

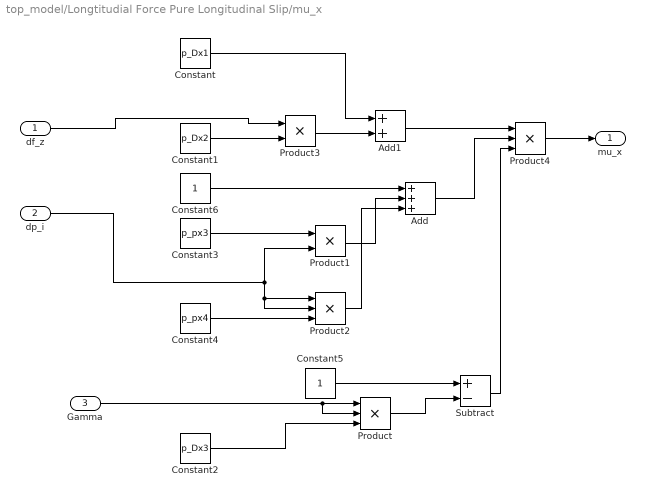
== system top_model/Longtitudial Force Pure Longitudinal Slip/mu_x ==
  df_z : Inport
  dp_i : Inport  Port=2
  Gamma : Inport  Port=3
  Add : Sum  Inputs=3
  Add1 : Sum
  Constant : Constant  Value=p_Dx1
  Constant1 : Constant  Value=p_Dx2
  Constant2 : Constant  Value=p_Dx3
  Constant3 : Constant  Value=p_px3
  Constant4 : Constant  Value=p_px4
  Constant5 : Constant
  Constant6 : Constant
  Product : Product  Inputs=3
  Product1 : Product
  Product2 : Product  Inputs=3
  Product3 : Product
  Product4 : Product  Inputs=3
  Subtract : Sum  Inputs=+-
  mu_x : Outport
  wires:
  Gamma/1 -> Product/2, Product/1
  Constant2/1 -> Product/3
  Constant5/1 -> Subtract/1
  Product/1 -> Subtract/2
  Constant3/1 -> Product1/1
  dp_i/1 -> Product2/1, Product2/2, Product1/2
  Constant4/1 -> Product2/3
  Constant6/1 -> Add/1
  Product1/1 -> Add/2
  Product2/1 -> Add/3
  Constant1/1 -> Product3/2
  df_z/1 -> Product3/1
  Product3/1 -> Add1/2
  Constant/1 -> Add1/1
  Add1/1 -> Product4/1
  Add/1 -> Product4/2
  Subtract/1 -> Product4/3
  Product4/1 -> mu_x/1
